simulink model "quadrotor_stage11_cbf"  (R2026a)
settings: Solver=ode4  StartTime=0  StopTime=30  FixedStep=0.005  MaxStep=0.005  RelTol=1e-6
undefined symbols (not defined in the file or in its folder): DiscIntNeverNeededParam
settings Model: Creator=ASUS  LastModifiedBy=ASUS

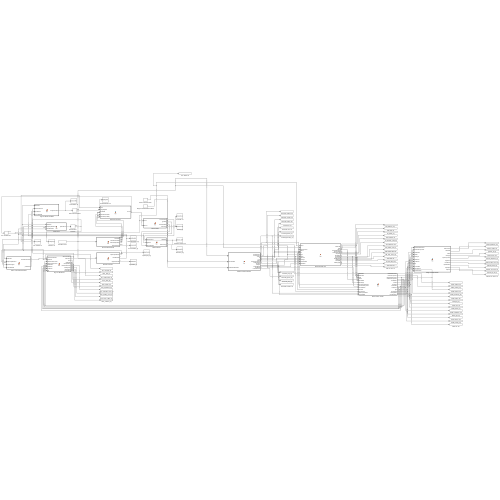
[thumbnail: Simulink's stored preview of the top-level diagram]
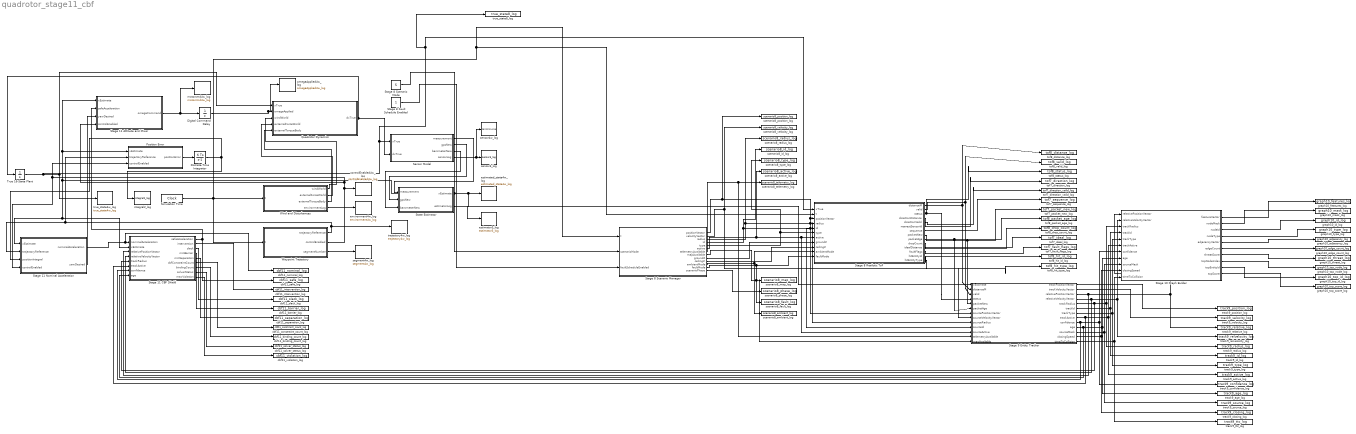
== system quadrotor_stage11_cbf ==
  Digital Command Delay : UnitDelay  InitialCondition=sqrt(1.20*9.81/(4*1.8e-5))*ones(4,1)  SampleTime=0.005
  Discrete-Time Integrator : DiscreteIntegrator  InitialCondition=zeros(3,1)  SampleTime=0.005  LimitOutput=on  UpperSaturationLimit=[4;4;1.5]  LowerSaturationLimit=[-4;-4;-1.5]  ICPrevOutput=DiscIntNeverNeededParam  ICPrevScaledInput=DiscIntNeverNeededParam
  Position Error : MATLAB Function  TreatAsAtomicUnit=on
  Quadrotor Dynamics : MATLAB Function  TreatAsAtomicUnit=on
  Sensor Model : MATLAB Function  TreatAsAtomicUnit=on
  Simulation Time : DigitalClock
  Stage 10 Graph Builder : MATLAB Function  TreatAsAtomicUnit=on
  Stage 11 Attitude and Mixer : MATLAB Function  TreatAsAtomicUnit=on
  Stage 11 CBF Shield : MATLAB Function  TreatAsAtomicUnit=on
  Stage 11 Nominal Acceleration : MATLAB Function  TreatAsAtomicUnit=on
  Stage 8 Fault Schedule Enabled : Constant
  Stage 8 Realistic ToF : MATLAB Function  TreatAsAtomicUnit=on
  Stage 8 Scenario Manager : MATLAB Function  TreatAsAtomicUnit=on
  Stage 8 Scenario Mode : Constant  Value=5
  Stage 9 Entity Tracker : MATLAB Function  TreatAsAtomicUnit=on
  State Estimator : MATLAB Function  TreatAsAtomicUnit=on
  True 16-State Plant : Integrator  InitialCondition=[zeros(12,1); sqrt(1.20*9.81/(4*1.8e-5))*ones(4,1)]
  Waypoint Trajectory : MATLAB Function  TreatAsAtomicUnit=on
  Wind and Disturbances : MATLAB Function  TreatAsAtomicUnit=on
  cbf11_barrier_log : ToWorkspace  VariableName=cbf11_barrier_log  SaveFormat=Timeseries  SampleTime=-1
      settings: Save2DSignal=2-D array (concatenate along first dimension)
  cbf11_binding_count_log : ToWorkspace  VariableName=cbf11_binding_count_log  SaveFormat=Timeseries  SampleTime=-1
      settings: Save2DSignal=2-D array (concatenate along first dimension)
  cbf11_constraint_count_log : ToWorkspace  VariableName=cbf11_constraint_count_log  SaveFormat=Timeseries  SampleTime=-1
      settings: Save2DSignal=2-D array (concatenate along first dimension)
  cbf11_intervention_log : ToWorkspace  VariableName=cbf11_intervention_log  SaveFormat=Timeseries  SampleTime=-1
      settings: Save2DSignal=2-D array (concatenate along first dimension)
  cbf11_nominal_log : ToWorkspace  VariableName=cbf11_nominal_log  SaveFormat=Timeseries  SampleTime=-1
      settings: Save2DSignal=2-D array (concatenate along first dimension)
  cbf11_safe_log : ToWorkspace  VariableName=cbf11_safe_log  SaveFormat=Timeseries  SampleTime=-1
      settings: Save2DSignal=2-D array (concatenate along first dimension)
  cbf11_separation_log : ToWorkspace  VariableName=cbf11_separation_log  SaveFormat=Timeseries  SampleTime=-1
      settings: Save2DSignal=2-D array (concatenate along first dimension)
  cbf11_slack_log : ToWorkspace  VariableName=cbf11_slack_log  SaveFormat=Timeseries  SampleTime=-1
      settings: Save2DSignal=2-D array (concatenate along first dimension)
  cbf11_solver_status_log : ToWorkspace  VariableName=cbf11_solver_status_log  SaveFormat=Timeseries  SampleTime=-1
      settings: Save2DSignal=2-D array (concatenate along first dimension)
  cbf11_violation_log : ToWorkspace  VariableName=cbf11_violation_log  SaveFormat=Timeseries  SampleTime=-1
      settings: Save2DSignal=2-D array (concatenate along first dimension)
  controlEnabled4w_log : ToWorkspace  VariableName=controlEnabled4w_log  SaveFormat=Timeseries  SampleTime=-1
      settings: Save2DSignal=2-D array (concatenate along first dimension)
  environment4w_log : ToWorkspace  VariableName=environment4w_log  SaveFormat=Timeseries  SampleTime=-1
      settings: Save2DSignal=2-D array (concatenate along first dimension)
  estimated_state4w_log : ToWorkspace  VariableName=estimated_state4w_log  SaveFormat=Timeseries  SampleTime=-1
      settings: Save2DSignal=2-D array (concatenate along first dimension)
  estimator3_log : ToWorkspace  VariableName=estimator3_log  SaveFormat=Timeseries  SampleTime=-1
      settings: Save2DSignal=2-D array (concatenate along first dimension)
  graph10_adjacency_log : ToWorkspace  VariableName=graph10_adjacency_log  SaveFormat=Timeseries  SampleTime=-1
      settings: Save2DSignal=2-D array (concatenate along first dimension)
  graph10_edge_count_log : ToWorkspace  VariableName=graph10_edge_count_log  SaveFormat=Timeseries  SampleTime=-1
      settings: Save2DSignal=2-D array (concatenate along first dimension)
  graph10_features_log : ToWorkspace  VariableName=graph10_features_log  SaveFormat=Timeseries  SampleTime=-1
      settings: Save2DSignal=2-D array (concatenate along first dimension)
  graph10_id_log : ToWorkspace  VariableName=graph10_id_log  SaveFormat=Timeseries  SampleTime=-1
      settings: Save2DSignal=2-D array (concatenate along first dimension)
  graph10_mask_log : ToWorkspace  VariableName=graph10_mask_log  SaveFormat=Timeseries  SampleTime=-1
      settings: Save2DSignal=2-D array (concatenate along first dimension)
  graph10_threat_log : ToWorkspace  VariableName=graph10_threat_log  SaveFormat=Timeseries  SampleTime=-1
      settings: Save2DSignal=2-D array (concatenate along first dimension)
  graph10_top_id_log : ToWorkspace  VariableName=graph10_top_id_log  SaveFormat=Timeseries  SampleTime=-1
      settings: Save2DSignal=2-D array (concatenate along first dimension)
  graph10_top_node_log : ToWorkspace  VariableName=graph10_top_node_log  SaveFormat=Timeseries  SampleTime=-1
      settings: Save2DSignal=2-D array (concatenate along first dimension)
  graph10_top_score_log : ToWorkspace  VariableName=graph10_top_score_log  SaveFormat=Timeseries  SampleTime=-1
      settings: Save2DSignal=2-D array (concatenate along first dimension)
  graph10_type_log : ToWorkspace  VariableName=graph10_type_log  SaveFormat=Timeseries  SampleTime=-1
      settings: Save2DSignal=2-D array (concatenate along first dimension)
  integral2_log : ToWorkspace  VariableName=integral2_log  SaveFormat=Timeseries  SampleTime=-1
      settings: Save2DSignal=2-D array (concatenate along first dimension)
  motorcmd4w_log : ToWorkspace  VariableName=motorcmd4w_log  SaveFormat=Timeseries  SampleTime=-1
      settings: Save2DSignal=2-D array (concatenate along first dimension)
  omegaApplied4w_log : ToWorkspace  VariableName=omegaApplied4w_log  SaveFormat=Timeseries  SampleTime=-1
      settings: Save2DSignal=2-D array (concatenate along first dimension)
  scenario8_active_log : ToWorkspace  VariableName=scenario8_active_log  SaveFormat=Timeseries  SampleTime=-1
      settings: Save2DSignal=2-D array (concatenate along first dimension)
  scenario8_ambient_log : ToWorkspace  VariableName=scenario8_ambient_log  SaveFormat=Timeseries  SampleTime=-1
      settings: Save2DSignal=2-D array (concatenate along first dimension)
  scenario8_fault_log : ToWorkspace  VariableName=scenario8_fault_log  SaveFormat=Timeseries  SampleTime=-1
      settings: Save2DSignal=2-D array (concatenate along first dimension)
  scenario8_id_log : ToWorkspace  VariableName=scenario8_id_log  SaveFormat=Timeseries  SampleTime=-1
      settings: Save2DSignal=2-D array (concatenate along first dimension)
  scenario8_map_log : ToWorkspace  VariableName=scenario8_map_log  SaveFormat=Timeseries  SampleTime=-1
      settings: Save2DSignal=2-D array (concatenate along first dimension)
  scenario8_phase_log : ToWorkspace  VariableName=scenario8_phase_log  SaveFormat=Timeseries  SampleTime=-1
      settings: Save2DSignal=2-D array (concatenate along first dimension)
  scenario8_position_log : ToWorkspace  VariableName=scenario8_position_log  SaveFormat=Timeseries  SampleTime=-1
      settings: Save2DSignal=2-D array (concatenate along first dimension)
  scenario8_radius_log : ToWorkspace  VariableName=scenario8_radius_log  SaveFormat=Timeseries  SampleTime=-1
      settings: Save2DSignal=2-D array (concatenate along first dimension)
  scenario8_telemetry_log : ToWorkspace  VariableName=scenario8_telemetry_log  SaveFormat=Timeseries  SampleTime=-1
      settings: Save2DSignal=2-D array (concatenate along first dimension)
  scenario8_type_log : ToWorkspace  VariableName=scenario8_type_log  SaveFormat=Timeseries  SampleTime=-1
      settings: Save2DSignal=2-D array (concatenate along first dimension)
  scenario8_velocity_log : ToWorkspace  VariableName=scenario8_velocity_log  SaveFormat=Timeseries  SampleTime=-1
      settings: Save2DSignal=2-D array (concatenate along first dimension)
  segment4w_log : ToWorkspace  VariableName=segment4w_log  SaveFormat=Timeseries  SampleTime=-1
      settings: Save2DSignal=2-D array (concatenate along first dimension)
  sensor3_log : ToWorkspace  VariableName=sensor3_log  SaveFormat=Timeseries  SampleTime=-1
      settings: Save2DSignal=2-D array (concatenate along first dimension)
  sensor4w_log : ToWorkspace  VariableName=sensor4w_log  SaveFormat=Timeseries  SampleTime=-1
      settings: Save2DSignal=2-D array (concatenate along first dimension)
  tof7_direction_log : ToWorkspace  VariableName=tof7_direction_log  SaveFormat=Timeseries  SampleTime=-1
      settings: Save2DSignal=2-D array (concatenate along first dimension)
  tof7_direction_valid_log : ToWorkspace  VariableName=tof7_direction_valid_log  SaveFormat=Timeseries  SampleTime=-1
      settings: Save2DSignal=2-D array (concatenate along first dimension)
  tof7_fault_flags_log : ToWorkspace  VariableName=tof7_fault_flags_log  SaveFormat=Timeseries  SampleTime=-1
      settings: Save2DSignal=2-D array (concatenate along first dimension)
  tof7_ideal_log : ToWorkspace  VariableName=tof7_ideal_log  SaveFormat=Timeseries  SampleTime=-1
      settings: Save2DSignal=2-D array (concatenate along first dimension)
  tof7_packet_new_log : ToWorkspace  VariableName=tof7_packet_new_log  SaveFormat=Timeseries  SampleTime=-1
      settings: Save2DSignal=2-D array (concatenate along first dimension)
  tof7_sequence_log : ToWorkspace  VariableName=tof7_sequence_log  SaveFormat=Timeseries  SampleTime=-1
      settings: Save2DSignal=2-D array (concatenate along first dimension)
  "tof8_distance_log    " : ToWorkspace  VariableName=tof8_distance_log  SaveFormat=Timeseries  SampleTime=-1
      settings: Save2DSignal=2-D array (concatenate along first dimension)
  tof8_drop_count_log : ToWorkspace  VariableName=tof8_drop_count_log  SaveFormat=Timeseries  SampleTime=-1
      settings: Save2DSignal=2-D array (concatenate along first dimension)
  tof8_hit_id_log : ToWorkspace  VariableName=tof8_hit_id_log  SaveFormat=Timeseries  SampleTime=-1
      settings: Save2DSignal=2-D array (concatenate along first dimension)
  tof8_hit_type_log : ToWorkspace  VariableName=tof8_hit_type_log  SaveFormat=Timeseries  SampleTime=-1
      settings: Save2DSignal=2-D array (concatenate along first dimension)
  tof8_packet_age_log : ToWorkspace  VariableName=tof8_packet_age_log  SaveFormat=Timeseries  SampleTime=-1
      settings: Save2DSignal=2-D array (concatenate along first dimension)
  "tof8_status_log " : ToWorkspace  VariableName=tof8_status_log  SaveFormat=Timeseries  SampleTime=-1
      settings: Save2DSignal=2-D array (concatenate along first dimension)
  tof8_valid_log : ToWorkspace  VariableName=tof8_valid_log  SaveFormat=Timeseries  SampleTime=-1
      settings: Save2DSignal=2-D array (concatenate along first dimension)
  track9_active_log : ToWorkspace  VariableName=track9_active_log  SaveFormat=Timeseries  SampleTime=-1
      settings: Save2DSignal=2-D array (concatenate along first dimension)
  track9_age_log : ToWorkspace  VariableName=track9_age_log  SaveFormat=Timeseries  SampleTime=-1
      settings: Save2DSignal=2-D array (concatenate along first dimension)
  track9_closing_log : ToWorkspace  VariableName=track9_closing_log  SaveFormat=Timeseries  SampleTime=-1
      settings: Save2DSignal=2-D array (concatenate along first dimension)
  track9_confidence_log : ToWorkspace  VariableName=track9_confidence_log  SaveFormat=Timeseries  SampleTime=-1
      settings: Save2DSignal=2-D array (concatenate along first dimension)
  track9_id_log : ToWorkspace  VariableName=track9_id_log  SaveFormat=Timeseries  SampleTime=-1
      settings: Save2DSignal=2-D array (concatenate along first dimension)
  track9_position_log : ToWorkspace  VariableName=track9_position_log  SaveFormat=Timeseries  SampleTime=-1
      settings: Save2DSignal=2-D array (concatenate along first dimension)
  track9_radius_log : ToWorkspace  VariableName=track9_radius_log  SaveFormat=Timeseries  SampleTime=-1
      settings: Save2DSignal=2-D array (concatenate along first dimension)
  track9_relative_log : ToWorkspace  VariableName=track9_relative_log  SaveFormat=Timeseries  SampleTime=-1
      settings: Save2DSignal=2-D array (concatenate along first dimension)
  track9_relvelocity_log : ToWorkspace  VariableName=track9_relvelocity_log  SaveFormat=Timeseries  SampleTime=-1
      settings: Save2DSignal=2-D array (concatenate along first dimension)
  track9_source_log : ToWorkspace  VariableName=track9_source_log  SaveFormat=Timeseries  SampleTime=-1
      settings: Save2DSignal=2-D array (concatenate along first dimension)
  track9_ttc_log : ToWorkspace  VariableName=track9_ttc_log  SaveFormat=Timeseries  SampleTime=-1
      settings: Save2DSignal=2-D array (concatenate along first dimension)
  track9_type_log : ToWorkspace  VariableName=track9_type_log  SaveFormat=Timeseries  SampleTime=-1
      settings: Save2DSignal=2-D array (concatenate along first dimension)
  track9_velocity_log : ToWorkspace  VariableName=track9_velocity_log  SaveFormat=Timeseries  SampleTime=-1
      settings: Save2DSignal=2-D array (concatenate along first dimension)
  trajectory4w_log : ToWorkspace  VariableName=trajectory4w_log  SaveFormat=Timeseries  SampleTime=-1
      settings: Save2DSignal=2-D array (concatenate along first dimension)
  true_state4w_log : ToWorkspace  VariableName=true_state4w_log  SaveFormat=Timeseries  SampleTime=-1
      settings: Save2DSignal=2-D array (concatenate along first dimension)
  true_state8_log : ToWorkspace  VariableName=true_state8_log  SaveFormat=Timeseries  SampleTime=-1
      settings: Save2DSignal=2-D array (concatenate along first dimension)
  wires:
  Stage 11 Attitude and Mixer/1(omegaCommand) -> motorcmd4w_log/1, Digital Command Delay/1
  True 16-State Plant/1 -> Sensor Model/1(xTrue), Stage 8 Realistic ToF/1(xTrue), true_state8_log/1, true_state4w_log/1, Quadrotor Dynamics/1(xTrue)
  Position Error/1(positionError) -> Discrete-Time Integrator/1
  Discrete-Time Integrator/1 -> Stage 11 Nominal Acceleration/3(positionIntegral), integral2_log/1
  Simulation Time/1 -> Waypoint Trajectory/1(t), Stage 8 Realistic ToF/2(t), Stage 8 Scenario Manager/1(t), Wind and Disturbances/1(t)
  Wind and Disturbances/1(windWorld) -> Quadrotor Dynamics/3(windWorld)
  Wind and Disturbances/2(externalForceWorld) -> Quadrotor Dynamics/4(externalForceWorld)
  Wind and Disturbances/3(externalTorqueBody) -> Quadrotor Dynamics/5(externalTorqueBody)
  Wind and Disturbances/4(environmentLog) -> environment4w_log/1
  Quadrotor Dynamics/1(dxTrue) -> True 16-State Plant/1, Sensor Model/2(dxTrue)
  Sensor Model/1(measurement) -> State Estimator/1(measurement)
  Sensor Model/2(gpsNew) -> State Estimator/2(gpsNew)
  Sensor Model/3(barometerNew) -> State Estimator/3(barometerNew)
  State Estimator/1(xEstimate) -> Stage 9 Entity Tracker/1(xEstimate), estimated_state4w_log/1, Stage 11 Attitude and Mixer/1(xEstimate), Position Error/1(xEstimate), Stage 11 CBF Shield/2(xEstimate), Stage 11 Nominal Acceleration/1(xEstimate)
  Waypoint Trajectory/1(trajectoryReference) -> Stage 11 Nominal Acceleration/2(trajectoryReference), Position Error/2(trajectoryReference), trajectory4w_log/1
  Waypoint Trajectory/2(controlEnabled) -> Stage 11 Nominal Acceleration/4(controlEnabled), Position Error/3(controlEnabled), Stage 11 Attitude and Mixer/4(controlEnabled), controlEnabled4w_log/1
  Digital Command Delay/1 -> omegaApplied4w_log/1, Quadrotor Dynamics/2(omegaApplied)
  State Estimator/2(estimatorLog) -> estimator3_log/1
  Sensor Model/4(sensorLog) -> sensor4w_log/1, sensor3_log/1
  Waypoint Trajectory/3(segmentNumber) -> segment4w_log/1
  Stage 8 Realistic ToF/1(distanceM) -> Stage 9 Entity Tracker/2(distanceM), "tof8_distance_log    "/1
  Stage 8 Realistic ToF/2(valid) -> Stage 9 Entity Tracker/3(valid), tof8_valid_log/1
  Stage 8 Realistic ToF/3(status) -> Stage 9 Entity Tracker/4(status), "tof8_status_log "/1
  Stage 8 Realistic ToF/4(directionDistance) -> tof7_direction_log/1
  Stage 8 Realistic ToF/5(directionValid) -> tof7_direction_valid_log/1
  Stage 8 Realistic ToF/7(sequence) -> tof7_sequence_log/1
  Stage 8 Realistic ToF/8(packetNew) -> Stage 9 Entity Tracker/5(packetNew), tof7_packet_new_log/1
  Stage 8 Realistic ToF/9(packetAge) -> tof8_packet_age_log/1, Stage 9 Entity Tracker/6(packetAge)
  Stage 8 Realistic ToF/10(dropCount) -> tof8_drop_count_log/1
  Stage 8 Realistic ToF/11(idealDistance) -> tof7_ideal_log/1
  Stage 8 Realistic ToF/12(faultFlags) -> tof7_fault_flags_log/1
  Stage 8 Scenario Mode/1 -> Stage 8 Scenario Manager/2(scenarioMode)
  Stage 8 Fault Schedule Enabled/1 -> Stage 8 Scenario Manager/3(faultScheduleEnabled)
  Stage 8 Realistic ToF/13(hitEntityId) -> tof8_hit_id_log/1
  Stage 8 Realistic ToF/14(hitEntityType) -> tof8_hit_type_log/1
  Stage 8 Scenario Manager/13(scenarioPhase) -> scenario8_phase_log/1
  Stage 8 Scenario Manager/7(telemetryAvailable) -> scenario8_telemetry_log/1, Stage 9 Entity Tracker/12(telemetryAvailable)
  Stage 8 Scenario Manager/2(velocityVector) -> Stage 9 Entity Tracker/8(sourceVelocityVector), scenario8_velocity_log/1
  Stage 8 Scenario Manager/6(active) -> scenario8_active_log/1, Stage 8 Realistic ToF/7(active), Stage 9 Entity Tracker/11(sourceActive)
  Stage 8 Scenario Manager/3(radius) -> scenario8_radius_log/1, Stage 9 Entity Tracker/9(sourceRadius), Stage 8 Realistic ToF/4(radius)
  Stage 8 Scenario Manager/4(id) -> scenario8_id_log/1, Stage 9 Entity Tracker/10(sourceId), Stage 8 Realistic ToF/5(id)
  Stage 8 Scenario Manager/1(positionVector) -> scenario8_position_log/1, Stage 9 Entity Tracker/7(sourcePositionVector), Stage 8 Realistic ToF/3(positionVector)
  Stage 8 Scenario Manager/11(ambientMode) -> scenario8_ambient_log/1, Stage 8 Realistic ToF/10(ambientMode)
  Stage 8 Scenario Manager/12(faultMode) -> scenario8_fault_log/1, Stage 8 Realistic ToF/11(faultMode)
  Stage 8 Scenario Manager/5(type) -> scenario8_type_log/1, Stage 8 Realistic ToF/6(type)
  Stage 8 Scenario Manager/9(groundZ) -> Stage 8 Realistic ToF/8(groundZ)
  Stage 8 Scenario Manager/8(mapAvailable) -> Stage 9 Entity Tracker/13(mapAvailable), scenario8_map_log/1
  Stage 8 Scenario Manager/10(ceilingZ) -> Stage 8 Realistic ToF/9(ceilingZ)
  Stage 9 Entity Tracker/1(trackPositionVector) -> track9_position_log/1
  Stage 9 Entity Tracker/2(trackVelocityVector) -> track9_velocity_log/1
  Stage 9 Entity Tracker/3(relativePositionVector) -> Stage 11 CBF Shield/3(relativePositionVector), Stage 10 Graph Builder/1(relativePositionVector), track9_relative_log/1
  Stage 9 Entity Tracker/4(relativeVelocityVector) -> Stage 11 CBF Shield/4(relativeVelocityVector), Stage 10 Graph Builder/2(relativeVelocityVector), track9_relvelocity_log/1
  Stage 9 Entity Tracker/5(trackRadius) -> Stage 11 CBF Shield/5(trackRadius), track9_radius_log/1, Stage 10 Graph Builder/3(trackRadius)
  Stage 9 Entity Tracker/6(trackId) -> track9_id_log/1, Stage 10 Graph Builder/4(trackId)
  Stage 9 Entity Tracker/7(trackType) -> track9_type_log/1, Stage 10 Graph Builder/5(trackType)
  Stage 9 Entity Tracker/8(trackActive) -> Stage 11 CBF Shield/6(trackActive), track9_active_log/1, Stage 10 Graph Builder/6(trackActive)
  Stage 9 Entity Tracker/9(confidence) -> track9_confidence_log/1, Stage 10 Graph Builder/7(confidence), Stage 11 CBF Shield/7(confidence)
  Stage 9 Entity Tracker/10(age) -> track9_age_log/1, Stage 10 Graph Builder/8(age), Stage 11 CBF Shield/8(age)
  Stage 9 Entity Tracker/11(sourceMask) -> track9_source_log/1, Stage 10 Graph Builder/9(sourceMask)
  Stage 9 Entity Tracker/12(closingSpeed) -> track9_closing_log/1, Stage 10 Graph Builder/10(closingSpeed)
  Stage 9 Entity Tracker/13(timeToCollision) -> track9_ttc_log/1, Stage 10 Graph Builder/11(timeToCollision)
  Stage 10 Graph Builder/1(featureVector) -> graph10_features_log/1
  Stage 10 Graph Builder/2(nodeMask) -> graph10_mask_log/1
  Stage 10 Graph Builder/3(nodeId) -> graph10_id_log/1
  Stage 10 Graph Builder/4(nodeType) -> graph10_type_log/1
  Stage 10 Graph Builder/5(adjacencyVector) -> graph10_adjacency_log/1
  Stage 10 Graph Builder/6(edgeCount) -> graph10_edge_count_log/1
  Stage 10 Graph Builder/7(threatScore) -> graph10_threat_log/1
  Stage 10 Graph Builder/8(topNodeIndex) -> graph10_top_node_log/1
  Stage 10 Graph Builder/9(topEntityId) -> graph10_top_id_log/1
  Stage 10 Graph Builder/10(topScore) -> graph10_top_score_log/1
  Stage 11 Nominal Acceleration/1(nominalAcceleration) -> cbf11_nominal_log/1, Stage 11 CBF Shield/1(nominalAcceleration)
  Stage 11 CBF Shield/1(safeAcceleration) -> cbf11_safe_log/1, Stage 11 Attitude and Mixer/2(safeAcceleration)
  Stage 11 Nominal Acceleration/2(yawDesired) -> Stage 11 Attitude and Mixer/3(yawDesired)
  Stage 11 CBF Shield/2(intervention) -> cbf11_intervention_log/1
  Stage 11 CBF Shield/3(slack) -> cbf11_slack_log/1
  Stage 11 CBF Shield/4(minBarrier) -> cbf11_barrier_log/1
  Stage 11 CBF Shield/5(minSeparation) -> cbf11_separation_log/1
  Stage 11 CBF Shield/6(cbfConstraintCount) -> cbf11_constraint_count_log/1
  Stage 11 CBF Shield/7(bindingCount) -> cbf11_binding_count_log/1
  Stage 11 CBF Shield/8(solverStatus) -> cbf11_solver_status_log/1
  Stage 11 CBF Shield/9(maxViolation) -> cbf11_violation_log/1

== matlab function quadrotor_stage11_cbf/Stage 9 Entity Tracker ==
  settings: updateMethod=DISCRETE  sampleTime=0.05
  data: xEstimate input; trackPositionVector output; distanceM input; valid input; status input; packetNew input; packetAge input; sourcePositionVector input; sourceVelocityVector input; sourceRadius input; sourceId input; sourceActive input; telemetryAvailable input; mapAvailable input; trackVelocityVector output; relativePositionVector output; relativeVelocityVector output; trackRadius output; trackId output; trackType output; trackActive output; confidence output; age output; sourceMask output; closingSpeed output; timeToCollision output
function [trackPositionVector,trackVelocityVector,relativePositionVector, ...
    relativeVelocityVector,trackRadius,trackId,trackType,trackActive, ...
    confidence,age,sourceMask,closingSpeed,timeToCollision] = ...
    fcn(xEstimate,distanceM,valid,status,packetNew,packetAge, ...
    sourcePositionVector,sourceVelocityVector,sourceRadius,sourceId, ...
    sourceActive,telemetryAvailable,mapAvailable)
%#codegen

trackPositionVector = zeros(48,1);
trackVelocityVector = zeros(48,1);
relativePositionVector = zeros(48,1);
relativeVelocityVector = zeros(48,1);
trackRadius = zeros(16,1);
trackId = zeros(16,1);
trackType = zeros(16,1);
trackActive = false(16,1);
confidence = zeros(16,1);
age = zeros(16,1);
sourceMask = zeros(16,1);
closingSpeed = zeros(16,1);
timeToCollision = 1000*ones(16,1);

allowedPosition = reshape(sourcePositionVector,3,16);
allowedVelocity = reshape(sourceVelocityVector,3,16);
allowedRadius = sourceRadius;
allowedId = sourceId;

% Remove unavailable ground truth before calling the tracker.
allowedActive = false(16,1);
for k = 1:16
    allowed = sourceActive(k) && ...
        (telemetryAvailable(k) || mapAvailable(k));
    allowedActive(k) = allowed;
    if ~allowed
        allowedPosition(:,k) = zeros(3,1);
        allowedVelocity(:,k) = zeros(3,1);
        allowedRadius(k) = 0.0;
        allowedId(k) = 0.0;
    end
end

[p,v,rp,rv,radius,id,type,active,conf,trackAge,mask,closing,ttc] = ...
    entityTrackerStage9(xEstimate,distanceM,valid,status,packetNew, ...
    packetAge,allowedPosition,allowedVelocity,allowedRadius,allowedId, ...
    allowedActive,telemetryAvailable,mapAvailable);

trackPositionVector(:) = reshape(p,48,1);
trackVelocityVector(:) = reshape(v,48,1);
relativePositionVector(:) = reshape(rp,48,1);
relativeVelocityVector(:) = reshape(rv,48,1);
trackRadius(:)=radius(:); trackId(:)=id(:); trackType(:)=type(:);
trackActive(:)=active(:); confidence(:)=conf(:); age(:)=trackAge(:);
sourceMask(:)=mask(:); closingSpeed(:)=closing(:);
timeToCollision(:)=ttc(:);
end

== matlab function quadrotor_stage11_cbf/Stage 10 Graph Builder ==
  settings: updateMethod=DISCRETE  sampleTime=0.10
  data: relativePositionVector input; featureVector output; relativeVelocityVector input; trackRadius input; trackId input; trackType input; trackActive input; confidence input; age input; sourceMask input; closingSpeed input; timeToCollision input; nodeMask output; nodeId output; nodeType output; adjacencyVector output; edgeCount output; threatScore output; topNodeIndex output; topEntityId output; topScore output
function [featureVector,nodeMask,nodeId,nodeType,adjacencyVector, ...
    edgeCount,threatScore,topNodeIndex,topEntityId,topScore] = ...
    fcn(relativePositionVector,relativeVelocityVector,trackRadius, ...
    trackId,trackType,trackActive,confidence,age,sourceMask, ...
    closingSpeed,timeToCollision)
%#codegen

featureVector = zeros(323,1);
nodeMask = false(17,1);
nodeId = zeros(17,1);
nodeType = zeros(17,1);
adjacencyVector = false(289,1);
edgeCount = 0.0;
threatScore = zeros(17,1);
topNodeIndex = zeros(5,1);
topEntityId = zeros(5,1);
topScore = zeros(5,1);

relativePosition = reshape(relativePositionVector,3,16);
relativeVelocity = reshape(relativeVelocityVector,3,16);

[features,mask,id,type,adjacency,edges,score,topNode,topId,rankedScore] = ...
    graphBuilderStage10(relativePosition,relativeVelocity,trackRadius, ...
    trackId,trackType,trackActive,confidence,age,sourceMask, ...
    closingSpeed,timeToCollision);

featureVector(:) = reshape(features,323,1);
nodeMask(:) = mask(:);
nodeId(:) = id(:);
nodeType(:) = type(:);
adjacencyVector(:) = reshape(adjacency,289,1);
edgeCount = edges;
threatScore(:) = score(:);
topNodeIndex(:) = topNode(:);
topEntityId(:) = topId(:);
topScore(:) = rankedScore(:);
end

== matlab function quadrotor_stage11_cbf/Stage 8 Scenario Manager ==
  settings: updateMethod=DISCRETE  sampleTime=0.05
  data: t input; positionVector output; scenarioMode input; faultScheduleEnabled input; velocityVector output; radius output; id output; type output; active output; telemetryAvailable output; mapAvailable output; groundZ output; ceilingZ output; ambientMode output; faultMode output; scenarioPhase output
function [positionVector,velocityVector,radius,id,type,active, ...
    telemetryAvailable,mapAvailable,groundZ,ceilingZ, ...
    ambientMode,faultMode,scenarioPhase] = ...
    fcn(t,scenarioMode,faultScheduleEnabled)
%#codegen

positionVector = zeros(48,1);
velocityVector = zeros(48,1);
radius = zeros(16,1);
id = zeros(16,1);
type = zeros(16,1);
active = false(16,1);
telemetryAvailable = false(16,1);
mapAvailable = false(16,1);
groundZ = 0.0;
ceilingZ = 2.5;
ambientMode = 0.0;
faultMode = 0.0;
scenarioPhase = 0.0;

[p,v,r,i,ty,a,telemetry,map,g,c,ambient,fault,phase] = ...
    skyGraphScenarioStage8(t(1),scenarioMode(1), ...
    faultScheduleEnabled(1));

positionVector(:) = reshape(p,48,1);
velocityVector(:) = reshape(v,48,1);
radius(:) = r(:);
id(:) = i(:);
type(:) = ty(:);
active(:) = a(:);
telemetryAvailable(:) = telemetry(:);
mapAvailable(:) = map(:);
groundZ = g;
ceilingZ = c;
ambientMode = ambient;
faultMode = fault;
scenarioPhase = phase;
end

== matlab function quadrotor_stage11_cbf/Stage 11 Nominal Acceleration ==
  settings: updateMethod=DISCRETE  sampleTime=0.05
  data: xEstimate input; nominalAcceleration output; trajectoryReference input; positionIntegral input; controlEnabled input; yawDesired output
function [nominalAcceleration,yawDesired] = ...
    fcn(xEstimate,trajectoryReference,positionIntegral,controlEnabled)
%#codegen
nominalAcceleration=zeros(3,1);
yawDesired=0.0;
[nominalAcceleration,yawDesired]=nominalAccelerationStage11( ...
    xEstimate,trajectoryReference,positionIntegral,controlEnabled);
end

== matlab function quadrotor_stage11_cbf/Stage 11 Attitude and Mixer ==
  settings: updateMethod=DISCRETE  sampleTime=0.005
  data: xEstimate input; omegaCommand output; safeAcceleration input; yawDesired input; controlEnabled input
function omegaCommand = ...
    fcn(xEstimate,safeAcceleration,yawDesired,controlEnabled)
%#codegen
omegaCommand=zeros(4,1);
omegaCommand=attitudeMotorControllerStage11( ...
    xEstimate,safeAcceleration,yawDesired,controlEnabled);
end

== matlab function quadrotor_stage11_cbf/Stage 11 CBF Shield ==
  settings: updateMethod=DISCRETE  sampleTime=0.05
  data: nominalAcceleration input; safeAcceleration output; xEstimate input; relativePositionVector input; relativeVelocityVector input; trackRadius input; trackActive input; confidence input; age input; intervention output; slack output; minBarrier output; minSeparation output; cbfConstraintCount output; bindingCount output; solverStatus output; maxViolation output
function [safeAcceleration,intervention,slack,minBarrier,minSeparation, ...
    cbfConstraintCount,bindingCount,solverStatus,maxViolation] = ...
    fcn(nominalAcceleration,xEstimate,relativePositionVector, ...
    relativeVelocityVector,trackRadius,trackActive,confidence,age)
%#codegen

safeAcceleration=zeros(3,1);
intervention=false;
slack=0.0;
minBarrier=100.0;
minSeparation=100.0;
cbfConstraintCount=0.0;
bindingCount=0.0;
solverStatus=0.0;
maxViolation=0.0;

relativePosition=reshape(relativePositionVector,3,16);
relativeVelocity=reshape(relativeVelocityVector,3,16);
egoVelocity=[xEstimate(4);xEstimate(5);xEstimate(6)];

[safeAcceleration,intervention,slack,minBarrier,minSeparation, ...
    cbfConstraintCount,bindingCount,solverStatus,maxViolation] = ...
    cbfSafetyShieldStage11(nominalAcceleration,egoVelocity, ...
    relativePosition,relativeVelocity,trackRadius,trackActive, ...
    confidence,age);
end

== matlab function quadrotor_stage11_cbf/Quadrotor Dynamics ==
  data: xTrue input; dxTrue output; omegaApplied input; windWorld input; externalForceWorld input; externalTorqueBody input
function dxTrue = fcn(xTrue, omegaApplied, windWorld, ...
    externalForceWorld, externalTorqueBody)
%#codegen

dxTrue = zeros(16,1);

dxTrue = quadDynamicsStage3( ...
    xTrue, omegaApplied, windWorld, ...
    externalForceWorld, externalTorqueBody);
end

== matlab function quadrotor_stage11_cbf/Position Error ==
  settings: updateMethod=DISCRETE  sampleTime=0.005
  data: xEstimate input; positionError output; trajectoryReference input; controlEnabled input
function positionError = fcn(xEstimate, trajectoryReference, controlEnabled)
%#codegen

positionError = zeros(3,1);
if controlEnabled(1)
    positionError(1) = trajectoryReference(1)-xEstimate(1);
    positionError(2) = trajectoryReference(2)-xEstimate(2);
    positionError(3) = trajectoryReference(3)-xEstimate(3);
end
end

== matlab function quadrotor_stage11_cbf/Wind and Disturbances ==
  data: t input; windWorld output; externalForceWorld output; externalTorqueBody output; environmentLog output
function [windWorld, externalForceWorld, ...
    externalTorqueBody, environmentLog] = fcn(t)
%#codegen

windWorld = zeros(3,1);
externalForceWorld = zeros(3,1);
externalTorqueBody = zeros(3,1);
environmentLog = zeros(9,1);
end

== matlab function quadrotor_stage11_cbf/Waypoint Trajectory ==
  data: t input; trajectoryReference output; controlEnabled output; segmentNumber output
function [trajectoryReference, controlEnabled, segmentNumber] = fcn(t)
%#codegen

trajectoryReference = zeros(10,1);
controlEnabled = false;
segmentNumber = 0.0;

[generatedReference, generatedEnable, generatedSegment] = ...
    waypointTrajectoryStage4(t(1));

trajectoryReference(1:10) = generatedReference(1:10);
controlEnabled = generatedEnable(1);
segmentNumber = generatedSegment(1);
end

== matlab function quadrotor_stage11_cbf/Sensor Model ==
  settings: updateMethod=DISCRETE  sampleTime=0.005
  data: xTrue input; measurement output; dxTrue input; gpsNew output; barometerNew output; sensorLog output
function [measurement, gpsNew, barometerNew, sensorLog] = ...
    fcn(xTrue, dxTrue)
%#codegen
[measurement, gpsNew, barometerNew, sensorLog] = ...
    sensorModelStage3(xTrue, dxTrue);
end

== matlab function quadrotor_stage11_cbf/State Estimator ==
  settings: updateMethod=DISCRETE  sampleTime=0.005
  data: measurement input; xEstimate output; gpsNew input; barometerNew input; estimatorLog output
function [xEstimate, estimatorLog] = ...
    fcn(measurement, gpsNew, barometerNew)
%#codegen

[xEstimate, estimatorLog] = stateEstimatorStage3( ...
    measurement, gpsNew, barometerNew);
end

== matlab function quadrotor_stage11_cbf/Stage 8 Realistic ToF ==
  settings: updateMethod=DISCRETE  sampleTime=0.05
  data: xTrue input; distanceM output; t input; positionVector input; radius input; id input; type input; active input; groundZ input; ceilingZ input; ambientMode input; faultMode input; valid output; status output; directionDistance output; directionValid output; nearestSensorId output; sequence output; packetNew output; packetAge output; dropCount output; idealDistance output; faultFlags output; hitEntityId output; hitEntityType output
function [distanceM,valid,status,directionDistance,directionValid, ...
    nearestSensorId,sequence,packetNew,packetAge,dropCount, ...
    idealDistance,faultFlags,hitEntityId,hitEntityType] = ...
    fcn(xTrue,t,positionVector,radius,id,type,active, ...
    groundZ,ceilingZ,ambientMode,faultMode)
%#codegen

distanceM = zeros(10,1);
valid = false(10,1);
status = zeros(10,1);
directionDistance = zeros(6,1);
directionValid = false(6,1);
nearestSensorId = -ones(6,1);
sequence = 0.0;
packetNew = false;
packetAge = 0.0;
dropCount = 0.0;
idealDistance = zeros(10,1);
faultFlags = 0.0;
hitEntityId = zeros(10,1);
hitEntityType = zeros(10,1);

position = reshape(positionVector,3,16);
[d,v,s,dd,dv,ns,seq,isNew,age,drops,ideal,flags,hitId,hitType] = ...
    realisticScenarioToFStage8(xTrue,t(1),position,radius,id,type, ...
    active,groundZ(1),ceilingZ(1),ambientMode(1),faultMode(1));

distanceM(:)=d(:); valid(:)=v(:); status(:)=s(:);
directionDistance(:)=dd(:); directionValid(:)=dv(:);
nearestSensorId(:)=ns(:); sequence=seq; packetNew=isNew;
packetAge=age; dropCount=drops; idealDistance(:)=ideal(:);
faultFlags=flags; hitEntityId(:)=hitId(:); hitEntityType(:)=hitType(:);
end
